simulink model "ModelloSimulink"  (R2020b)
settings: Solver=VariableStepAuto  StartTime=0.0  StopTime=10.0  RelTol=1e-3
values from neighbouring files (symbols this model uses):
  C = minreal((1/Gzas)* (Gcl/ (1- Gcl)))    [parte2.m]
  C2 = minreal((1/Gzas)* (Gcl2/ (1- Gcl2)))    [parte2.m]
  Gzas = tf(10, conv([1 -0.1],[1 -0.8]), Tc)    [parte2.m]
  Tc = 0.1    [parte2.m]
settings Model: Creator=chiar  LastModifiedBy=chiar

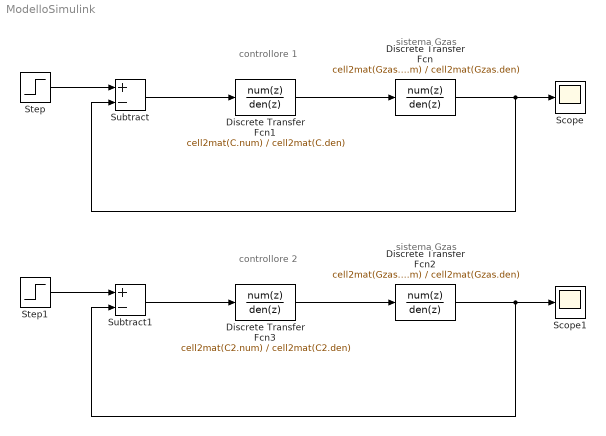
== system ModelloSimulink ==
  note: controllore 1
  note: sistema Gzas
  note: controllore 2
  note: sistema Gzas
  Discrete Transfer Fcn : DiscreteTransferFcn  Numerator=cell2mat(Gzas.num)  Denominator=cell2mat(Gzas.den)  SampleTime=Tc
  Discrete Transfer Fcn1 : DiscreteTransferFcn  Numerator=cell2mat(C.num)  Denominator=cell2mat(C.den)  SampleTime=Tc
  Discrete Transfer Fcn2 : DiscreteTransferFcn  Numerator=cell2mat(Gzas.num)  Denominator=cell2mat(Gzas.den)  SampleTime=Tc
  Discrete Transfer Fcn3 : DiscreteTransferFcn  Numerator=cell2mat(C2.num)  Denominator=cell2mat(C2.den)  SampleTime=Tc
  Scope : Scope
  Scope1 : Scope
  Step : Step  SampleTime=0
  Step1 : Step  SampleTime=0
  Subtract : Sum  Inputs=+-
  Subtract1 : Sum  Inputs=+-
  wires:
  Step/1 -> Subtract/1
  Subtract/1 -> Discrete Transfer Fcn1/1
  Discrete Transfer Fcn1/1 -> Discrete Transfer Fcn/1
  Discrete Transfer Fcn/1 -> Subtract/2, Scope/1
  Step1/1 -> Subtract1/1
  Discrete Transfer Fcn2/1 -> Subtract1/2, Scope1/1
  Discrete Transfer Fcn3/1 -> Discrete Transfer Fcn2/1
  Subtract1/1 -> Discrete Transfer Fcn3/1
